simulink model "SIMULINK_RSED_MODEL"  (R2020b)
settings: Solver=FixedStepAuto  StartTime=0.0  StopTime=inf  RelTol=1e-3  EnableMultiTasking=on
settings Model: SILPILModeSetting=veronly  ExtModeTrigDuration=2  Creator=tcbir  LastModifiedBy=tcbir
settings OptimizationCC: EnhancedBackFolding=on  PassReuseOutputArgsAs=Individual arguments  ZeroExternalMemoryAtStartup=off  ZeroInternalMemoryAtStartup=off  MaxStackSize=64  OptimizeBlockOrder=speed  DifferentSizesBufferReuse=on  OptimizationCustomize=off  EfficientTunableParamExpr=on
settings DebuggingCC: ParameterTunabilityLossMsg=error
settings HardwareCC: ProdBitPerInt=16  ProdBitPerPointer=16  ProdBitPerSizeT=16  ProdBitPerPtrDiffT=16  ProdLargestAtomicFloat=None  ProdWordSize=8  ProdHWDeviceType=Atmel->AVR  UseEmbeddedCoderFeatures=off  UseSimulinkCoderFeatures=off
settings SFSimCC: MATLABDynamicMemAlloc=off
settings RTWCC: Description=Embedded Coder  SystemTargetFile=ert.tlc  HardwareBoard=Arduino Mega 2560  TemplateMakefile=ert_default_tmf  Toolchain=Arduino AVR  BuildConfiguration=Faster Runs
settings CodeAppCC: ForceParamTrailComments=on  IgnoreCustomStorageClasses=off  OperatorAnnotations=on  SimulinkDataObjDesc=on  SFDataObjDesc=on  InsertBlockDesc=on
settings ERTTargetCC: SupportContinuousTime=on  SupportNonInlinedSFcns=on  SupportVariableSizeSignals=on  ExtModeStaticAllocSize=2048

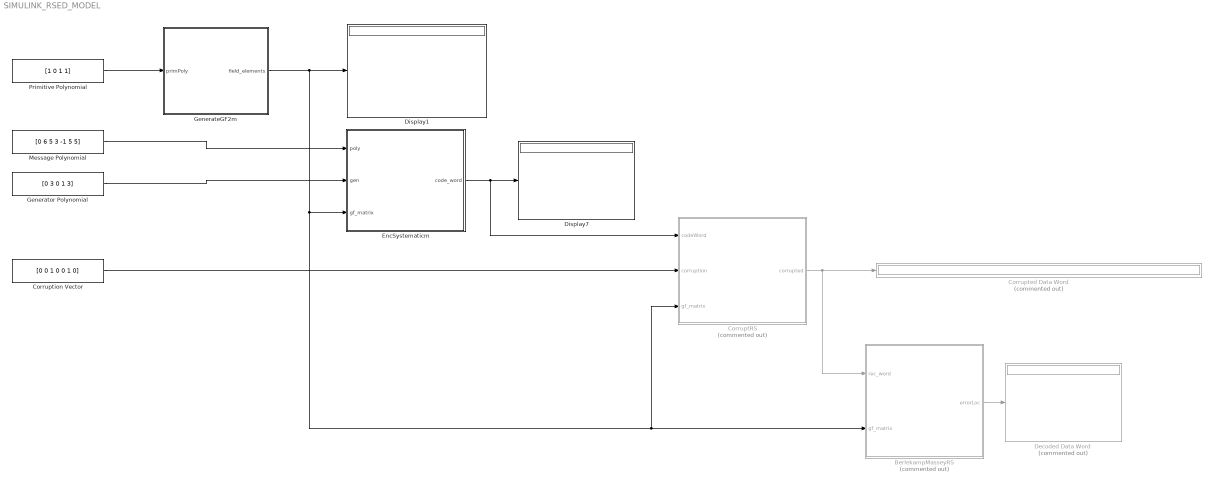
== system SIMULINK_RSED_MODEL ==
  BerlekampMasseyRS : MATLAB Function  Commented=on  TreatAsAtomicUnit=on
  CorruptRS : MATLAB Function  Commented=on  TreatAsAtomicUnit=on
  Corrupted Data Word : Display  Commented=on
  Corruption Vector : Constant  Value=[0 0 1 0 0 1 0]
  Decoded Data Word : Display  Commented=on
  Display1 : Display
  Display7 : Display
  EncSystematicm : MATLAB Function  TreatAsAtomicUnit=on
  GenerateGF2m : MATLAB Function  TreatAsAtomicUnit=on
  Generator Polynomial : Constant  Value=[0 3 0 1 3]
  Message Polynomial : Constant  Value=[0 6 5 3 -1 5 5]
  Primitive Polynomial : Constant  Value=[1 0 1 1]
  wires:
  CorruptRS/1(corrupted) -> BerlekampMasseyRS/1(rec_word), Corrupted Data Word/1
  GenerateGF2m/1(field_elements) -> BerlekampMasseyRS/2(gf_matrix), CorruptRS/3(gf_matrix), EncSystematicm/3(gf_matrix), Display1/1
  Corruption Vector/1 -> CorruptRS/2(corruption)
  BerlekampMasseyRS/1(errorLoc) -> Decoded Data Word/1
  Message Polynomial/1 -> EncSystematicm/1(poly)
  Generator Polynomial/1 -> EncSystematicm/2(gen)
  Primitive Polynomial/1 -> GenerateGF2m/1(primPoly)
  EncSystematicm/1(code_word) -> CorruptRS/1(codeWord), Display7/1

== matlab function SIMULINK_RSED_MODEL/CorruptRS ==
  data: codeWord input; corrupted output; corruption input; gf_matrix input
function corrupted  = CorruptRS(codeWord, corruption, gf_matrix)
%This function randomly corrupts bits in locations specified by the user
m = 2^numel(gf_matrix(1,:)) - 1;
for i= 1:numel(codeWord)
    if corruption(i) == 1
        codeWord(i) = randi([0,m - 1]);
    end
end
corrupted = codeWord;
end

== matlab function SIMULINK_RSED_MODEL/EncSystematicm ==
  data: poly input; code_word output; gen input; gf_matrix input
% Systematic Encoding Method
% 1. Creates a temporary code word 
% 2. Uses polynomial division to find the remainder
% 3. Creates the codeword through polynomial addition
% Inputs: Message polynomial, generatory polynomial, and gf_matrix
% Output: Returns codeword from using that method
% Example Input: EncSystematicm([0 4 2],[0 3 0 1 3],GenerateGF2m(3,[1 0 1 1]))

function code_word  = EncSystematicm(poly,gen,gf_matrix)
m = numel(gf_matrix(1,:));  % set m to number of rows (power of 2)
numShifts = (2^m) - 1; 
power = numShifts - m; % find power which is n-k


x = ones(1: power+1);
x(power+1) =0;
% ask dona
% Filling the rest of the polynomial with inf
for i = (power+1):-1:2
    x(i) = -1;
end
% 
% % Shifting the temp polynomial 
temp_cw = PolyMultGF2m(x,poly,gf_matrix);

% temp_cw/gen = remainder 
% get the remainder
[q,r] = PolyDivGF2m(temp_cw,gen,gf_matrix);

% if the remainder array is smaller than the codeword array
if(numel(temp_cw) > numel(r))
    % find the offset between the codeword - remainder array
    diff = numel(temp_cw) - numel(r);
    % for the number of offsets
    for i = 1:diff
        % add infs to the left of the array
        r = [-1, r(1:end-1)];
    end
end


code_word = -1*ones(1, numShifts);
% Create the actual codeword using addition
% iterate through each index backwards
for i = numShifts:-1:1
        code_word(i) = AddGF2m(temp_cw(i),r(i),gf_matrix);
end

== matlab function SIMULINK_RSED_MODEL/GenerateGF2m ==
  data: primPoly input; field_elements output
% GenerateGF2m: generates the selected Galois Field element. The inputs should be the
% order m and the coefficients of an appropriate primitive polynomial. The generated field,
% in either binary or power notation, may be a calling parameter for each of the other
% functions. Hint: I strongly suggest that you input the coefficients in “power” notation,
% with the highest order power on the left

function field_elements  = GenerateGF2m(primPoly) %primPoly in power notation, highest order on left

m = 3;
% hard coded size of retrun matrices and gf mtrix because simulink
% whines about variable output size. Havent figured out how to fix it
% ask laberge
gf = zeros(8, 3); %there are 2^m field elements
field_elements = zeros(8, 3); %there are 2^m field elements

gfIndx = 2; %gfIndx(1) holds initial state 
numShifts = (2^m) - 1;
s_reg = zeros(1,int8(m));
s_reg(end) = 1; %rightmost element of init shr is 1
gf(1, :) = 0;%write the contents of the init shift register to the matrix of gf elements
gf(2, :) = s_reg;
for i = 2:numShifts %number of shifts corresponds to power of primitive element
    carryOut = s_reg(1);%save the value to be wrapped
    for i0 = 1:numel(s_reg)-1
        if primPoly(i0 + 1) == 1
            s_reg(i0) = xor(carryOut, s_reg(i0 + 1));
        else
            s_reg(i0) = s_reg(i0 + 1);
        end
    end
    s_reg(end) = carryOut;
    gf(i+1,:) = s_reg; %add the newly shifted register to the gf matrix
end
field_elements = gf;
end

== matlab function SIMULINK_RSED_MODEL/BerlekampMasseyRS ==
  data: rec_word input; errorLoc output; gf_matrix input
%function [c_hat_RS,failure] = BerlekampMasseyRS(gf_matrix, rec_word)
%This function implements the Berlekamp-Massey Algorithm for determining
%the Error Locator Polynomial for a given code word.
%inputs: GF2m matrix with binary coefficients
%received word polynomial in power notation (powers of alpha)
%output: the corrected word in power notation
function errorLoc  = BerlekampMasseyRS(rec_word, gf_matrix)
%print = ['decoding ', num2str(rec_word(:).'), ' using Berlekamp-Massey Algorithm...'];
%disp(print);
m = numel(gf_matrix(1,:));
n = (2^m) - 1;
r = n - m;
decFail = 0; %indicates decoder failure

%step 1
%compute the syndromes S1...Sr for the received codeword and form the
%syndrome polynomial
syndromes = zeros(1, r); %holds syndrome polynomial in alpha power notation, [S(1)....S(r)] 
for i = 1:r
    syndromes(i) = EvalPolyGF2m(rec_word, i, gf_matrix); %calculate each syndrome
end

if syndromes(1:end) == -1 %if all syndromes are zero, no errors
%   disp('No errors found. Berlekamp-Massey complete.');
   return;
end

k = 0;
L = 0;
tx = [0 -1]; %x, highest power on left
lambdaK = -1*ones(1, n+1);
lambdaK(end) = 0; %x
lambdaKm1 = lambdaK;

    while k < r
        %step 3**************************************************
        k = k + 1;
        %compute the big sum
            %multiply the things
            step3sum = -1; %initialize the sum
            lambdaIndx = numel(lambdaKm1) - 1;
            for i = 1:L 
                in1 = lambdaKm1(lambdaIndx); %should be 0 then 2
                in2 = syndromes(k - i); %should be 2 then inf
                p = MultGF2m(in1, in2, gf_matrix); %multiply lambda(k-1)by the k-ith syndrome
            
                step3sum = AddGF2m(step3sum, p, gf_matrix); %add multiplication result to big sum
                lambdaIndx = lambdaIndx - 1;
            end 
            deltaK = AddGF2m(syndromes(k), step3sum, gf_matrix); %compute the discrepancy  
        %end step 3**********************************************************
      
        %step 4
        if deltaK == -1 %if deltaK == 0, step 8
            %step 8
            tx(numel(tx) + 1) = -1; %Shift T(x) to the left (higher power): T(x) = xT(x).
        else %otherwise step 5,6
            %step 5
            %modify connection polynomial
            product = PolyMultGF2m(deltaK, tx, gf_matrix);
            productIndx = numel(product);
            
            %figure out how many places there are to add
            if numel(product) < numel(lambdaKm1)
                numAdds = numel(product);
            else
                numAdds = numel(lambdaKm1);
            end
            
            lambdaK_i = numel(lambdaK); %we may need to have a temp array to store the addition if the product is longer than lambda. will this ever happen?
            for i1 = 1:numAdds %start from x^0 and move to higher powers adding each index
                lambdaK(lambdaK_i) = AddGF2m(lambdaKm1(lambdaK_i), product(productIndx), gf_matrix); 
                lambdaK_i = lambdaK_i - 1;
                productIndx = productIndx - 1;
            end
            %step 6
            if (2*L) >= k %if 2L>=k, step 8
                %step 8
                tx(numel(tx) + 1) = -1; %Shift T(x) to the left (higher power): T(x) = xT(x).            
            else %otherwise step 7 then step 8
                %step 7
                L = k - L;
                if lambdaKm1(1:end-1) == -1
                    tx = DivGF2m(lambdaKm1(end), deltaK, gf_matrix); %tx = delta(k-1)x/delta(k)
                else
                    tx = PolyDivGF2m(lambdaKm1, deltaK, gf_matrix); %tx = delta(k-1)x/delta(k)
                end
            
                %step 8
                tx(numel(tx) + 1) = -1; %Shift T(x) to the left (higher power): T(x) = xT(x).
            end
        end
        %update k - 1 variables
        lambdaKm1 = lambdaK;
        %deltaKm1 = deltaK;
    end
    
%     handle decoder failure
%     find the highest degree of lambda
%     degree = 0;
%     for i2 = 1:numel(lambdaK)
%         if lambdaK(i2) > degree && lambdaK(i2) ~= inf
%             degree = lambdaK(i2);
%         end
%     end
    i2 = numel(lambdaK);
    degree = -1; %to account for 0th degree
    while lambdaK(i2) ~= -1
        i2 = i2 - 1;
        degree = degree + 1;
    end
    
    %if degree > r %(r/2)
    %    decFail = 1;
    %    fail = '************DECODER FAILURE************';
    %    disp(fail);
    %end

    %step 10
    %the error locator polynomial is the result of step k
    errorLoc = lambdaK;
    %printres = ['the error locator polynomial is: ', num2str(errorLoc(:).'), '. Berlekamp-Massey complete.'];
    %disp(printres);
    
    if decFail == 0
        %run chien and forney
        chien = chienSearch(errorLoc, degree, gf_matrix);
        if chien ~= 'x' %if not decode failure
            forney = ForneyAlgorithmRS(lambdaK,syndromes,chien,gf_matrix);
            CorrectionRS(rec_word,forney, gf_matrix)
        end
    end
    
end
